simulink model "Sarah_Emily_OTRB"  (R2014a)
settings: Solver=ode3  StartTime=0.0  StopTime=5  FixedStep=.001  RelTol=1e-3
libraries: simulink x1
settings Model: Creator=sarahcostrell  LastModifiedBy=kothmann
settings DebuggingCC: MergeDetectMultiDrivingBlocksExec=error

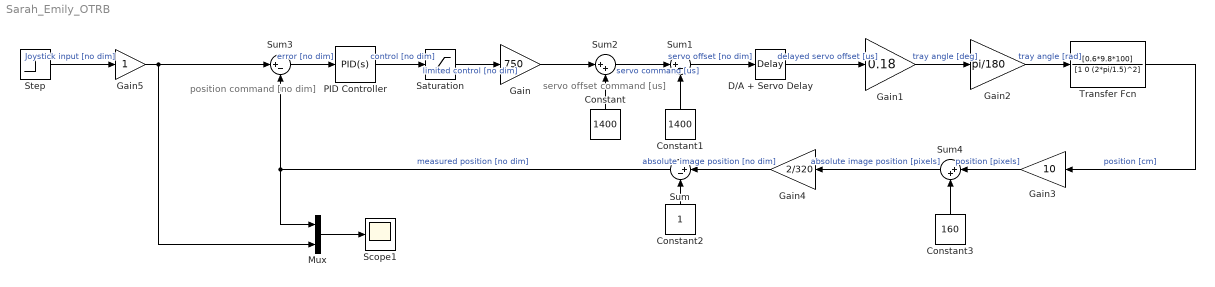
== system Sarah_Emily_OTRB ==
  note: position
      | command
      | [no dim]
  note: servo
      | offset
      | command
      | [us]
  Constant : Constant  Value=1400
  Constant1 : Constant  Value=1400
  Constant2 : Constant
  Constant3 : Constant  Value=160
  D/A + Servo Delay : TransportDelay  DelayTime=.08
  Gain : Gain  Gain=750
  Gain1 : Gain  Gain=0.18
  Gain2 : Gain  Gain=pi/180
  Gain3 : Gain  Gain=10
  Gain4 : Gain  Gain=2/320
  Gain5 : Gain
  Mux : Mux  Inputs=2
  PID Controller : simulink/Continuous/PID Controller  Controller=PID  TimeDomain=Continuous-time  SampleTime=-1  IntegratorMethod=Forward Euler  FilterMethod=Forward Euler  Form=Parallel  P=0.2  I=.2  D=.06  N=100  InitialConditionSource=internal  InitialConditionForIntegrator=0  InitialConditionForFilter=0  ExternalReset=none  LimitOutput=off  UpperSaturationLimit=inf  LowerSaturationLimit=-inf  LinearizeAsGain=on  AntiWindupMode=none  Kb=1  TrackingMode=off  Kt=1  PParamMin=[]  PParamMax=[]  IParamMin=[]  IParamMax=[]  DParamMin=[]  DParamMax=[]  NParamMin=[]  NParamMax=[]  KbParamMin=[]  KbParamMax=[]  KtParamMin=[]  KtParamMax=[]  POutMin=[]  POutMax=[]  IOutMin=[]  IOutMax=[]  DOutMin=[]  DOutMax=[]  NOutMin=[]  NOutMax=[]  KbOutMin=[]  KbOutMax=[]  KtOutMin=[]  KtOutMax=[]  IntegratorOutMin=[]  IntegratorOutMax=[]  FilterOutMin=[]  FilterOutMax=[]  SumOutMin=[]  SumOutMax=[]  SumI1OutMin=[]  SumI1OutMax=[]  SumI2OutMin=[]  SumI2OutMax=[]  SumI3OutMin=[]  SumI3OutMax=[]  SumDOutMin=[]  SumDOutMax=[]  SaturationOutMin=[]  SaturationOutMax=[]  IntegratorContinuousStateAttributes=''  IntegratorStateMustResolveToSignalObject=off  IntegratorRTWStateStorageClass=Auto  FilterContinuousStateAttributes=''  FilterStateMustResolveToSignalObject=off  FilterRTWStateStorageClass=Auto
  Saturation : Saturate
  Scope1 : Scope
      settings: TimeRange=5  YMin=0  YMax=0.25
  Step : Step  After=0.2  SampleTime=0
  Sum : Sum  Inputs=|+-
  Sum1 : Sum  Inputs=|+-
  Sum2 : Sum  Inputs=|++
  Sum3 : Sum  Inputs=|+-
  Sum4 : Sum  Inputs=|++
  Transfer Fcn : TransferFcn  Numerator=[0.6*9.8*100]  Denominator=[1 0 (2*pi/1.5)^2]
  wires:
  Sum1/1 -> D/A + Servo Delay/1  "servo offset [no dim]"
  Gain1/1 -> Gain2/1  "tray angle [deg]"
  Gain2/1 -> Transfer Fcn/1  "tray angle [rad]"
  Constant1/1 -> Sum1/2
  Constant/1 -> Sum2/2
  Gain/1 -> Sum2/1
  Sum2/1 -> Sum1/1  "servo command [us]"
  Gain4/1 -> Sum/1  "absolute image position [no dim]"
  Constant2/1 -> Sum/2
  PID Controller/1 -> Saturation/1  "control [no dim]"
  Sum3/1 -> PID Controller/1  "error [no dim]"
  Gain5/1 -> Mux/2, Sum3/1
  Step/1 -> Gain5/1  "Joystick input [no dim]"
  Saturation/1 -> Gain/1  "limited control [no dim]"
  Transfer Fcn/1 -> Gain3/1  "position [cm]"
  Constant3/1 -> Sum4/2
  Gain3/1 -> Sum4/1  "position [pixels]"
  D/A + Servo Delay/1 -> Gain1/1  "delayed servo offset [us]"
  Sum4/1 -> Gain4/1  "absolute image position [pixels]"
  Sum/1 -> Mux/1, Sum3/2  "measured position [no dim]"
  Mux/1 -> Scope1/1
